simulink model "Ejemplo3"  (Simulink 5.0)
settings: Solver=ode45  StartTime=0.0  StopTime=10.0  RelTol=1e-3
undefined symbols (not defined in the file or in its folder): k
settings Model: LastModifiedBy=gaby

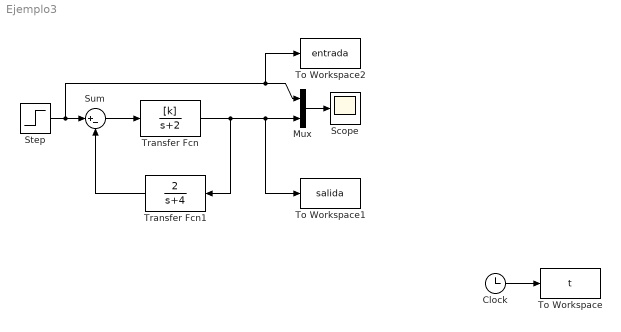
== system Ejemplo3 ==
  Clock : Clock
      settings: Decimation=10
  Mux : Mux  Inputs=2
  Scope : Scope
  Step : Step  SampleTime=0
  Sum : Sum  Inputs=|+-  SaturateOnIntegerOverflow=on
  To Workspace : ToWorkspace  VariableName=t  SampleTime=-1  SaveFormat=Array
  To Workspace1 : ToWorkspace  VariableName=salida  SampleTime=-1  SaveFormat=Array
  To Workspace2 : ToWorkspace  VariableName=entrada  SampleTime=-1  SaveFormat=Array
  Transfer Fcn : TransferFcn  Numerator=[k]  Denominator=[1 2]
  Transfer Fcn1 : TransferFcn  Orientation=left  Numerator=[2]  Denominator=[1 4]
  wires:
  Transfer Fcn/1 -> Transfer Fcn1/1, Mux/2, To Workspace1/1
  Transfer Fcn1/1 -> Sum/2
  Sum/1 -> Transfer Fcn/1
  Step/1 -> Sum/1, Mux/1, To Workspace2/1
  Mux/1 -> Scope/1
  Clock/1 -> To Workspace/1
